simulink model "fuzzy_controller"  (R2015a)
settings: Solver=ode45  StartTime=0.0  StopTime=10.0  RelTol=1e-3
libraries: fuzblock x2, simulink x1
settings Model: Creator=BML  LastModifiedBy=BML

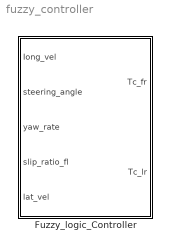
== system fuzzy_controller ==
  Fuzzy_logic_Controller : Subsystem

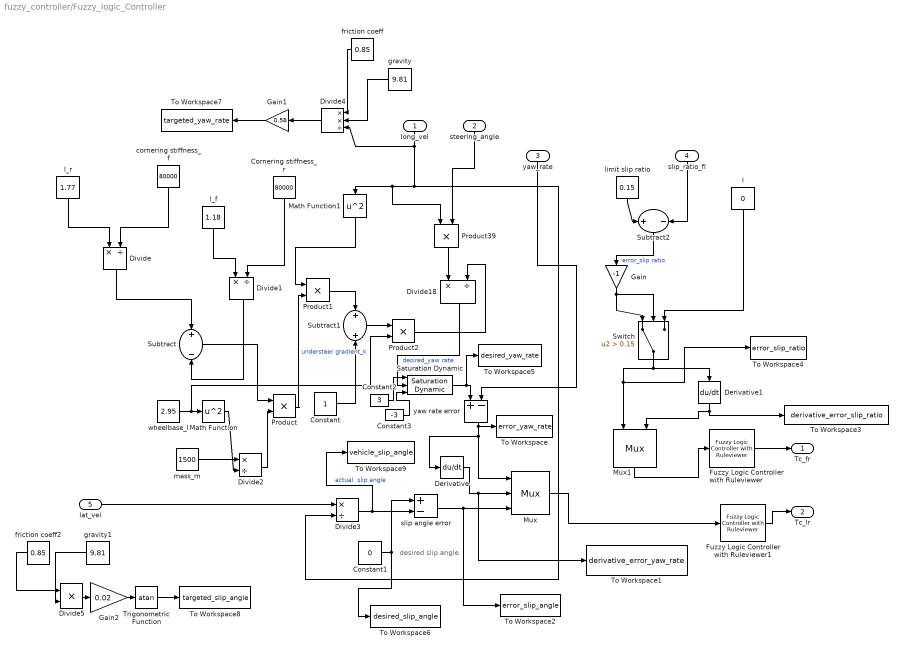
== system fuzzy_controller/Fuzzy_logic_Controller ==
  note: desired
      | slip angle
  Iong_vel : Inport
  steering_angle : Inport  Port=2
  yaw_rate : Inport  Port=3
  slip_ratio_fl : Inport  Port=4
  lat_vel : Inport  Port=5
  Constant : Constant
  Constant1 : Constant  Value=0
  Constant2 : Constant  Value=3
  Constant3 : Constant  Value=-3
  "Cornering stiffness_r " : Constant  Value=80000
  Derivative : Derivative
  Derivative1 : Derivative
  Divide{,1..3,18} (5 alike) : Product  Inputs=*/
  Divide4 : Product  Inputs=**/
  Divide5 : Product  Inputs=**
  Fuzzy Logic Controller with Ruleviewer : fuzblock/Fuzzy Logic  Controller  with Ruleviewer  fismatrix=fuzzy_slip_ratio1  Ts=2
  Fuzzy Logic Controller with Ruleviewer1 : fuzblock/Fuzzy Logic  Controller  with Ruleviewer  fismatrix=fuzzy_yaw_rate1  Ts=2
  Gain : Gain  Gain=-1
  Gain1 : Gain  Gain=0.58
  Gain2 : Gain  Gain=0.02
  Math Function : Math  Operator=square  SaturateOnIntegerOverflow=on
  Math Function1 : Math  Operator=square  SaturateOnIntegerOverflow=on
  Mux : Mux  Inputs=3
  Mux1 : Mux  Inputs=2
  Product{,1..2,39} (4 alike) : Product
  Saturation Dynamic : simulink/Discontinuities/Saturation Dynamic  OutMin=-3  OutMax=3  OutDataTypeStr=Inherit: Same as second input  OutDataType=fixdt(1, 16)  OutScaling=2^-10  DoSatur=off
  Subtract : Sum  Inputs=+-
  Subtract1 : Sum
  Subtract2 : Sum  Inputs=+-
  Switch : Switch  Criteria=u2 > Threshold  Threshold=0.15
  To Workspace : ToWorkspace  VariableName=error_yaw_rate  SaveFormat=Timeseries  SampleTime=1
  To Workspace1 : ToWorkspace  VariableName=derivative_error_yaw_rate  SaveFormat=Timeseries  SampleTime=1
  To Workspace2 : ToWorkspace  VariableName=error_slip_angle  SaveFormat=Timeseries  SampleTime=1
  To Workspace3 : ToWorkspace  VariableName=derivative_error_slip_ratio  SaveFormat=Timeseries  SampleTime=1
  To Workspace4 : ToWorkspace  VariableName=error_slip_ratio  SaveFormat=Timeseries  SampleTime=1
  To Workspace5 : ToWorkspace  VariableName=desired_yaw_rate  SaveFormat=Timeseries  SampleTime=1
  To Workspace6 : ToWorkspace  VariableName=desired_slip_angle  SaveFormat=Timeseries  SampleTime=1
  To Workspace7 : ToWorkspace  VariableName=targeted_yaw_rate  SaveFormat=Timeseries  SampleTime=1
  To Workspace8 : ToWorkspace  VariableName=targeted_slip_angle  SaveFormat=Timeseries  SampleTime=1
  To Workspace9 : ToWorkspace  VariableName=vehicle_slip_angle  SaveFormat=Timeseries  SampleTime=1
  Trigonometric Function : Trigonometry  Operator=atan
  "cornering stiffness_f " : Constant  Value=80000
  friction coeff : Constant  Value=0.85
  friction coeff2 : Constant  Value=0.85
  gravity : Constant  Value=9.81
  gravity1 : Constant  Value=9.81
  l : Constant  Value=0
  "l_f " : Constant  Value=1.18
  "l_r " : Constant  Value=1.77
  limit slip ratio : Constant  Value=0.15
  mass_m : Constant  Value=1500
  "slip angle error  " : Sum  Inputs=+-
  wheelbase_l : Constant  Value=2.95
  "yaw rate error   " : Sum  Inputs=+-
  Tc_fr : Outport
  Tc_lr : Outport  Port=2
  wires:
  Fuzzy Logic Controller with Ruleviewer/1 -> Tc_fr/1
  Divide/1 -> Subtract/1
  Subtract/1 -> Product/1
  Product/1 -> Product1/2  "understeer gradient_k"
  Constant/1 -> Subtract1/2
  Product39/1 -> Divide18/1
  Product2/1 -> Divide18/2
  steering_angle/1 -> Product39/2
  Math Function1/1 -> Product1/1
  Subtract1/1 -> Product2/1
  lat_vel/1 -> Divide3/1
  "l_r "/1 -> Divide/1
  Divide1/1 -> Subtract/2
  "Cornering stiffness_r "/1 -> Divide1/2
  wheelbase_l/1 -> Product2/2, Math Function/1
  mass_m/1 -> Divide2/1
  Math Function/1 -> Divide2/2
  Divide2/1 -> Product/2
  "l_f "/1 -> Divide1/1
  "cornering stiffness_f "/1 -> Divide/2
  Product1/1 -> Subtract1/1
  Switch/1 -> Mux1/1, To Workspace4/1, Derivative1/1
  yaw_rate/1 -> "yaw rate error   "/2
  Divide18/1 -> Saturation Dynamic/2  "desired_yaw rate"
  Subtract2/1 -> Gain/1  "error_slip ratio"
  limit slip ratio/1 -> Subtract2/1
  Derivative/1 -> To Workspace1/1, Mux/2
  Mux/1 -> Fuzzy Logic Controller with Ruleviewer1/1
  slip_ratio_fl/1 -> Subtract2/2
  Divide3/1 -> To Workspace9/1, "slip angle error  "/2  "actual  slip angle"
  "slip angle error  "/1 -> To Workspace2/1, Mux/3
  Derivative1/1 -> Mux1/2, To Workspace3/1
  Mux1/1 -> Fuzzy Logic Controller with Ruleviewer/1
  Fuzzy Logic Controller with Ruleviewer1/1 -> Tc_lr/1
  "yaw rate error   "/1 -> To Workspace/1, Mux/1, Derivative/1
  Constant1/1 -> "slip angle error  "/1, To Workspace6/1
  friction coeff/1 -> Divide4/1
  Iong_vel/1 -> Divide3/2, Math Function1/1, Product39/1, Divide4/3
  gravity/1 -> Divide4/2
  Divide4/1 -> Gain1/1
  Gain1/1 -> To Workspace7/1
  friction coeff2/1 -> Divide5/1
  gravity1/1 -> Divide5/2
  Divide5/1 -> Gain2/1
  Gain2/1 -> Trigonometric Function/1
  Trigonometric Function/1 -> To Workspace8/1
  l/1 -> Switch/3
  Gain/1 -> Switch/1, Switch/2
  Constant2/1 -> Saturation Dynamic/1
  Constant3/1 -> Saturation Dynamic/3
  Saturation Dynamic/1 -> To Workspace5/1, "yaw rate error   "/1
